simulink subsystem "PieroAJModel"  (R2023b)
settings: Solver=VariableStepAuto  StartTime=0.0  StopTime=10.0  RelTol=1e-3
settings Model: Creator=jaime  LastModifiedBy=jaime

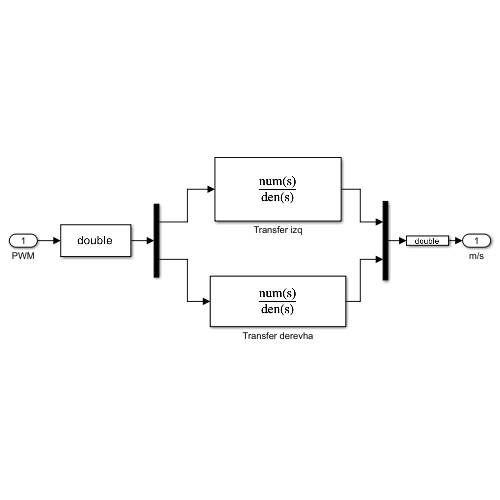
[thumbnail: Simulink's stored preview of the top-level diagram]
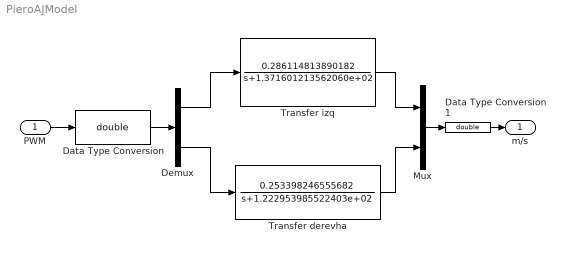
== system PieroAJModel ==
  PWM : Inport
  Data Type Conversion : DataTypeConversion  OutDataTypeStr=double  SaturateOnIntegerOverflow=off  RndMeth=Floor
  Data Type Conversion1 : DataTypeConversion  OutDataTypeStr=double  SaturateOnIntegerOverflow=off  RndMeth=Floor
  Demux : Demux  Outputs=2
  Mux : Mux  Inputs=2
  Transfer derevha : TransferFcn  Numerator=0.253398246555682  Denominator=[1,1.222953985522403e+02]
  Transfer izq : TransferFcn  Numerator=0.286114813890182  Denominator=[1,1.371601213562060e+02]
  m/s : Outport
  wires:
  PWM/1 -> Data Type Conversion/1
  Data Type Conversion/1 -> Demux/1
  Transfer derevha/1 -> Mux/2
  Demux/2 -> Transfer derevha/1
  Transfer izq/1 -> Mux/1
  Demux/1 -> Transfer izq/1
  Mux/1 -> Data Type Conversion1/1
  Data Type Conversion1/1 -> m/s/1
